simulink model "Diagrama_invernadero_industrial"  (R2019b)
settings: Solver=VariableStepAuto  StartTime=0.0  StopTime=24  RelTol=1e-3
libraries: Libreria x10
settings Model: Creator=PC-01  LastModifiedBy=PC-01

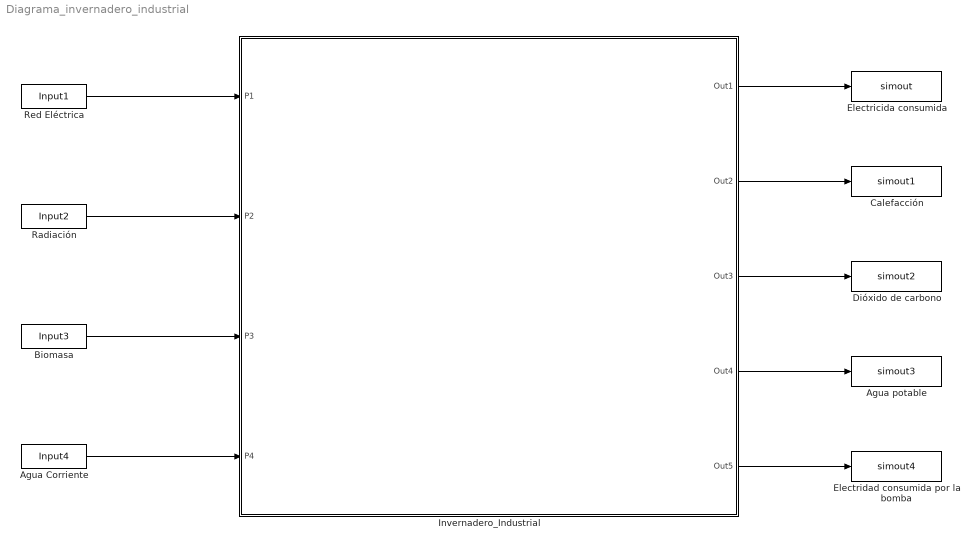
== system Diagrama_invernadero_industrial ==
  Agua Corriente : FromWorkspace  VariableName=Input4  SampleTime=0
  Agua potable : ToWorkspace  VariableName=simout3  SaveFormat=Timeseries  SampleTime=-1
  Biomasa : FromWorkspace  VariableName=Input3  SampleTime=0
  Calefacción : ToWorkspace  VariableName=simout1  SaveFormat=Timeseries  SampleTime=-1
  Dióxido de carbono : ToWorkspace  VariableName=simout2  SaveFormat=Timeseries  SampleTime=-1
  Electricida consumida : ToWorkspace  VariableName=simout  SaveFormat=Timeseries  SampleTime=-1
  Electridad consumida por la bomba : ToWorkspace  VariableName=simout4  SaveFormat=Timeseries  SampleTime=-1
  Invernadero_Industrial : Subsystem
  Radiación : FromWorkspace  VariableName=Input2  SampleTime=0
  Red Eléctrica : FromWorkspace  VariableName=Input1  SampleTime=0
  wires:
  Red Eléctrica/1 -> Invernadero_Industrial/1(P1)
  Radiación/1 -> Invernadero_Industrial/2(P2)
  Biomasa/1 -> Invernadero_Industrial/3(P3)
  Agua Corriente/1 -> Invernadero_Industrial/4(P4)
  Invernadero_Industrial/1(Out1) -> Electricida consumida/1
  Invernadero_Industrial/2(Out2) -> Calefacción/1
  Invernadero_Industrial/3(Out3) -> Dióxido de carbono/1
  Invernadero_Industrial/4(Out4) -> Agua potable/1
  Invernadero_Industrial/5(Out5) -> Electridad consumida por la bomba/1

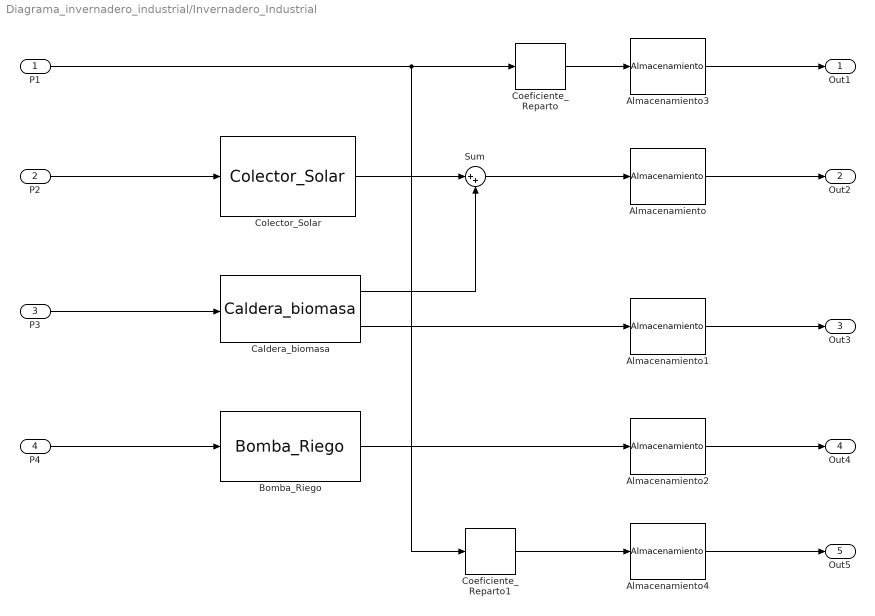
== system Diagrama_invernadero_industrial/Invernadero_Industrial ==
  P1 : Inport
  P2 : Inport  Port=2
  P3 : Inport  Port=3
  P4 : Inport  Port=4
  Almacenamiento : Libreria/Almacenamiento  Up2=1000  Low2=0  r_c=1  Up=1000  Low=0  r_d=1  Up1=1000  Low1=0  almacenamiento_inicial=0  cpa=0  almacenamiento_on=on
      link override In1: SampleTime=1
      link override Qch: VariableName=Qchp2
      link override Qdis: VariableName=Qdisp2
      link override ef: VariableName=Ech2
      link override eff: VariableName=Edis2
  Almacenamiento1 : Libreria/Almacenamiento  Up2=1000  Low2=0  r_c=1  Up=1000  Low=0  r_d=1  Up1=1000  Low1=0  almacenamiento_inicial=0  cpa=0  almacenamiento_on=on
      link override In1: SampleTime=1
      link override Qch: VariableName=Qchp3
      link override Qdis: VariableName=Qdisp3
      link override ef: VariableName=Ech3
      link override eff: VariableName=Edis3
  Almacenamiento2 : Libreria/Almacenamiento  Up2=1000  Low2=0  r_c=1  Up=1000  Low=0  r_d=1  Up1=1000  Low1=0  almacenamiento_inicial=0  cpa=0  almacenamiento_on=on
      link override In1: SampleTime=1
      link override Qch: VariableName=Qchp4
      link override Qdis: VariableName=Qdisp4
      link override ef: VariableName=Ech4
      link override eff: VariableName=Edis4
  Almacenamiento3 : Libreria/Almacenamiento  Up2=1000  Low2=0  r_c=1  Up=1000  Low=0  r_d=1  Up1=1000  Low1=0  almacenamiento_inicial=0  cpa=0  almacenamiento_on=on
      link override In1: SampleTime=1
      link override Qch: VariableName=Qchp1
      link override Qdis: VariableName=Qdisp1
      link override ef: VariableName=Ech1
      link override eff: VariableName=Edis1
  Almacenamiento4 : Libreria/Almacenamiento  Up2=1000  Low2=0  r_c=1  Up=1000  Low=0  r_d=1  Up1=1000  Low1=0  almacenamiento_inicial=0  cpa=1  almacenamiento_on=off
      link override In1: SampleTime=1
      link override Qch: VariableName=Qchp5
      link override Qdis: VariableName=Qdisp5
      link override ef: VariableName=Ech5
      link override eff: VariableName=Edis5
  Bomba_Riego : Libreria/Bomba_Riego  efficiency=1  dispatch_factor=beta1  T_muestreo=T_muestreo  Max_in=150  Max_out=150  n_salida=[5]
  Caldera_biomasa : Libreria/Caldera_biomasa  efficiency=[2 2]  dispatch_factor=1  T_muestreo=T_muestreo  Max_in=10000  Min_in=0  Max_out=[10000 10000]
  Coeficiente_Reparto : Libreria/Coeficiente_Reparto  dispatch_factor=alfa1  Tm=T_muestreo  Max_out=inf  Max_in=inf  efficiency=1
  Coeficiente_Reparto1 : Libreria/Coeficiente_Reparto  dispatch_factor=alfa2  Tm=T_muestreo  Max_out=inf  Max_in=inf  efficiency=1
  Colector_Solar : Libreria/Colector_Solar  efficiency=[0.211]  dispatch_factor=1  T_muestreo=T_muestreo  Max_in=1200  Max_out=2000
  Sum : Sum  Inputs=|++
  Out1 : Outport
  Out2 : Outport  Port=2
  Out3 : Outport  Port=3
  Out4 : Outport  Port=4
  Out5 : Outport  Port=5
  wires:
  Coeficiente_Reparto1/1 -> Almacenamiento4/1
  Sum/1 -> Almacenamiento/1
  Bomba_Riego/1 -> Almacenamiento2/1
  P1/1 -> Coeficiente_Reparto1/1, Coeficiente_Reparto/1
  P3/1 -> Caldera_biomasa/1
  Caldera_biomasa/1 -> Sum/2
  Colector_Solar/1 -> Sum/1
  Almacenamiento/1 -> Out2/1
  Caldera_biomasa/2 -> Almacenamiento1/1
  Coeficiente_Reparto/1 -> Almacenamiento3/1
  Almacenamiento1/1 -> Out3/1
  P4/1 -> Bomba_Riego/1
  P2/1 -> Colector_Solar/1
  Almacenamiento2/1 -> Out4/1
  Almacenamiento3/1 -> Out1/1
  Almacenamiento4/1 -> Out5/1
